simulink model "Ball_and_Plate_MicroLabBox_student"  (R2019b)
settings: Solver=ode1  StartTime=0.0  StopTime=Inf  FixedStep=0.001  RelTol=1e-3
PostLoadFcn:
  | , if any(exist('dsrtsu_mdlpostloadfcn', 'file') ~= 0), dsrtsu_mdlpostloadfcn('Execute', bdroot); end,
InitFcn:
  | , if any(exist('rtifpga_mdlclblib', 'file') ~= 0), rtifpga_mdlclblib('Init', bdroot); end,
values from neighbouring files (symbols this model uses):
  A_obs = A_fast - L*C_fast    [Init_workspace.m]
  B_obs = [B_fast, L]    [Init_workspace.m]
  C_obs = eye(4)    [Init_workspace.m]
  D_obs = zeros(4,4)    [Init_workspace.m]
  path = quintic(-0.0289,3,0,1/fs)    [Init_workspace.m]    (also in Quintic_Time.m = reference_end; Quintic_Velocity.m = reference_end)
  Ts_Outer = 0.1    [Init_workspace.m]
  uA = repmat(uA,[1,P])    [Init_workspace.m]
  uB = repmat(uB,[1,P])    [Init_workspace.m]
  uC = repmat(uC,[1,P])    [Init_workspace.m]
libraries: rtiemclib x6, rtiethernetlib x3, rti1202lib_dac_class1 x3, simulink x1
(part 3 of 3)

== matlab function Ball_and_Plate_MicroLabBox_student/Innerloop_Actuator/Motor_C/Init_motion/MATLAB Function1 ==
  data: reference_end input; path output; end_time input; Ts input; measured_position input
function path = Quintic_Polynomial_Trajectory_Time(reference_end, end_time, Ts, measured_position)
%% Quintic_Polynomial_Trajectory(reference_end, average_velocity)
% This function outputs a quintic polynomial trajectory over time in 
% Simulink given the end reference and average velocity. The starting 
% velocity and acceleration are set to zero.
%
% Input Arguments
% reference_end = desired end position of the trajectory
% end_time = end time of trajectory; for every new input 
% trajectory starts at time 0 and ends at end_time
% measured_position = current position of the robot arm
%
% Output Arguments
% path = path of the trajectory over time
%
% Quinten Swaan 17-08-2022
%
% Control Systems Technology group
% Departement of Mechanical Engineering
% Eindhoven University of Technology


persistent previous_value_reference_start previous_value_reference_end ...
    path_array index 

if isempty(previous_value_reference_start)
    previous_value_reference_start = 0;
end

if isempty(previous_value_reference_end)
    previous_value_reference_end = 0;
end

if isempty(path_array)
    path_array = zeros(1,1);
end

if isempty(index)
    index = 1;
end


% Obtain new trajectory if a new end reference is given
if previous_value_reference_end ~= reference_end
    t0 = 0;                                 %Starting time
    q0 = previous_value_reference_start;    %Starting position
    v0 = 0;                                 %Starting velocity
    ac0 = 0;                                %Starting acceleration
    tf = end_time;                          %End time
    qf = reference_end;                     %End position
    vf = 0;                                 %End velocity
    acf = 0;                                %End acceleration

    M = [1 t0 t0^2 t0^3 t0^4 t0^5;
    0 1 2*t0 3*t0^2 4*t0^3 5*t0^4;
    0 0 2 6*t0 12*t0^2 20*t0^3;
    1 tf tf^2 tf^3 tf^4 tf^5;
    0 1 2*tf 3*tf^2 4*tf^3 5*tf^4;
    0 0 2 6*tf 12*tf^2 20*tf^3];

    b = [q0; v0; ac0; qf; vf; acf];

    x = M \ b;

    t = t0:Ts:tf;

    path_array = x(1) + x(2).*t + x(3).*t.^2 + x(4).*t.^3 + +x(5).*t.^4 + x(6).*t.^5;

    index = 1;
    reference_current = path_array(index);

% Output the reference per timestep
else
    if index < length(path_array)
        index = index + 1;
    end
    reference_current = path_array(index);
end

previous_value_reference_end = reference_end;
previous_value_reference_start = measured_position;

path = reference_current;

== matlab function Ball_and_Plate_MicroLabBox_student/Innerloop_Actuator/Motor_C/Init_motion/MATLAB Function2 ==
  data: y input; path output; start input; init_value input; current_pos input
function path = init_motion(y, start, init_value, current_pos)

if start > 0.5
    path = init_value;
elseif start < 0.5
    path = y;
else 
    path = 0;
end

== matlab function Ball_and_Plate_MicroLabBox_student/Innerloop_Actuator/Motor_A/Init_motion/MATLAB Function ==
  data: enable input; u input; y output
function y = init_motion(enable, u)

persistent index previous_enable

% Initialize
if isempty(index)
    index = 1;
end

if isempty(previous_enable)
    previous_enable = 0;
end

N = length(u);

% Detect rising edge (re-enable)
if enable && ~previous_enable
    index = 1;
end

% Output logic
if enable

    % If still inside signal → output sample
    if index <= N
        y = u(index);
        index = index + 1;

    else
        % Signal finished → output zero
        y = 0;
    end

else
    % Disabled → output zero
    y = -0.0289;
end

previous_enable = enable;

== matlab function Ball_and_Plate_MicroLabBox_student/Innerloop_Actuator/Motor_B/Init_motion/MATLAB Function ==
  data: enable input; u input; y output
function y = init_motion(enable, u)

persistent index previous_enable

% Initialize
if isempty(index)
    index = 1;
end

if isempty(previous_enable)
    previous_enable = 0;
end

N = length(u);

% Detect rising edge (re-enable)
if enable && ~previous_enable
    index = 1;
end

% Output logic
if enable

    % If still inside signal → output sample
    if index <= N
        y = u(index);
        index = index + 1;

    else
        % Signal finished → output zero
        y = 0;
    end

else
    % Disabled → output zero
    y = -0.0289;
end

previous_enable = enable;

== matlab function Ball_and_Plate_MicroLabBox_student/Innerloop_Actuator/Motor_C/Init_motion/MATLAB Function ==
  data: enable input; u input; y output
function y = init_motion(enable, u)

persistent index previous_enable

% Initialize
if isempty(index)
    index = 1;
end

if isempty(previous_enable)
    previous_enable = 0;
end

N = length(u);

% Detect rising edge (re-enable)
if enable && ~previous_enable
    index = 1;
end

% Output logic
if enable

    % If still inside signal → output sample
    if index <= N
        y = u(index);
        index = index + 1;

    else
        % Signal finished → output zero
        y = 0;
    end

else
    % Disabled → output zero
    y = -0.0289;
end

previous_enable = enable;

== matlab function Ball_and_Plate_MicroLabBox_student/Innerloop_Actuator/AngleToPos  ==
  data: alpha input; pos1 output; beta input; psi input; pos2 output; pos3 output
function [pos1, pos2, pos3] = angleToPos(alpha, beta, psi)
    % Returns the actuator positions required to reach the desired angle
    % note: the position is absolute in the global frame

    % Physical Constants
    r = 0.17;           % Joint radius (m)
    T = [0; 0; 0.322];  % Resting height vector (m)
    
    % Joint positions on base and plate (equilateral triangle)
    % These match the definitions in your posToAngle function
    theta = [0, deg2rad(240), deg2rad(120)];
    B = [r*cos(theta); r*sin(theta); zeros(1,3)]; % Base joints (b_i)
    P = [r*cos(theta); r*sin(theta); zeros(1,3)]; % Plate joints (p_i)
    
    % Rotation Matrices (Yaw-Pitch-Roll order)
    Rz = [cos(psi) -sin(psi) 0; sin(psi) cos(psi) 0; 0 0 1];
    Ry = [cos(beta) 0 sin(beta); 0 1 0; -sin(beta) 0 cos(beta)];
    Rx = [1 0 0; 0 cos(alpha) -sin(alpha); 0 sin(alpha) cos(alpha)];
    R_BtoP = Rz * Ry * Rx; 
    
    % Compute absolute position for each motor
    % Motor 1
    l1_vec = T + (R_BtoP * P(:,1)) - B(:,1);
    pos1 = norm(l1_vec);
    
    % Motor 2
    l2_vec = T + (R_BtoP * P(:,2)) - B(:,2);
    pos2 = norm(l2_vec);
    
    % Motor 3
    l3_vec = T + (R_BtoP * P(:,3)) - B(:,3);
    pos3 = norm(l3_vec);
end

== matlab function Ball_and_Plate_MicroLabBox_student/Innerloop_Actuator/Motor_A/MATLAB Function1 ==
  data: reference_end input; path output; end_time input; Ts input; measured_position input
function path = Quintic_Time(reference_end, end_time, Ts, measured_position)
% QUINTIC_POLYNOMIAL_TRAJECTORY_TIME
% Calculated analytically per step to be compatible with dSPACE/Control Desk.

% Persistent variables to store coefficients and the "internal clock"
persistent coeffs t_elapsed prev_ref_end tf_internal
if isempty(coeffs)
    coeffs = zeros(6, 1); % a0, a1, a2, a3, a4, a5
end
if isempty(t_elapsed)
    t_elapsed = 0;
end
if isempty(prev_ref_end)
    prev_ref_end = reference_end;
end
if isempty(tf_internal)
    tf_internal = 0;
end

% Check if a new trajectory is requested
if reference_end ~= prev_ref_end
    % Reset timer
    t_elapsed = 0;
    tf_internal = end_time;
    
    % Boundary conditions
    q0 = prev_ref_end; 
    qf = reference_end;
    v0 = 0; vf = 0;
    ac0 = 0; acf = 0;
    
    % Solver for t0 = 0
    % We solve the system: M * coeffs = b
    % Using tf_internal instead of end_time to ensure consistency during the run
    T = tf_internal;
    M = [1, 0, 0,  0,    0,    0;
         0, 1, 0,  0,    0,    0;
         0, 0, 2,  0,    0,    0;
         1, T, T^2, T^3,  T^4,  T^5;
         0, 1, 2*T, 3*T^2, 4*T^3, 5*T^4;
         0, 0, 2,   6*T,   12*T^2, 20*T^3];
     
    b = [q0; v0; ac0; qf; vf; acf];
    
    % Calculate coefficients (Matrix is small 6x6, so this is fast)
    coeffs = M \ b;
end

% Calculate current reference based on elapsed time
t = t_elapsed;

if t <= tf_internal
    % Quintic Equation: path = a0 + a1*t + a2*t^2 + a3*t^3 + a4*t^4 + a5*t^5
    path = coeffs(1) + coeffs(2)*t + coeffs(3)*t^2 + coeffs(4)*t^3 + coeffs(5)*t^4 + coeffs(6)*t^5;
    
    % Increment time for the next step
    t_elapsed = t_elapsed + Ts;
else
    % Hold the final position once trajectory is finished
    path = reference_end;
end

% Update memory for next iteration
prev_ref_end = reference_end;

end

== matlab function Ball_and_Plate_MicroLabBox_student/Innerloop_Actuator/Motor_B/MATLAB Function2 ==
  data: reference_end input; path output; end_time input; Ts input; measured_position input
function path = Quintic_Time(reference_end, end_time, Ts, measured_position)
% QUINTIC_POLYNOMIAL_TRAJECTORY_TIME
% Calculated analytically per step to be compatible with dSPACE/Control Desk.

% Persistent variables to store coefficients and the "internal clock"
persistent coeffs t_elapsed prev_ref_end tf_internal
if isempty(coeffs)
    coeffs = zeros(6, 1); % a0, a1, a2, a3, a4, a5
end
if isempty(t_elapsed)
    t_elapsed = 0;
end
if isempty(prev_ref_end)
    prev_ref_end = reference_end;
end
if isempty(tf_internal)
    tf_internal = 0;
end

% Check if a new trajectory is requested
if reference_end ~= prev_ref_end
    % Reset timer
    t_elapsed = 0;
    tf_internal = end_time;
    
    % Boundary conditions
    q0 = prev_ref_end; 
    qf = reference_end;
    v0 = 0; vf = 0;
    ac0 = 0; acf = 0;
    
    % Solver for t0 = 0
    % We solve the system: M * coeffs = b
    % Using tf_internal instead of end_time to ensure consistency during the run
    T = tf_internal;
    M = [1, 0, 0,  0,    0,    0;
         0, 1, 0,  0,    0,    0;
         0, 0, 2,  0,    0,    0;
         1, T, T^2, T^3,  T^4,  T^5;
         0, 1, 2*T, 3*T^2, 4*T^3, 5*T^4;
         0, 0, 2,   6*T,   12*T^2, 20*T^3];
     
    b = [q0; v0; ac0; qf; vf; acf];
    
    % Calculate coefficients (Matrix is small 6x6, so this is fast)
    coeffs = M \ b;
end

% Calculate current reference based on elapsed time
t = t_elapsed;

if t <= tf_internal
    % Quintic Equation: path = a0 + a1*t + a2*t^2 + a3*t^3 + a4*t^4 + a5*t^5
    path = coeffs(1) + coeffs(2)*t + coeffs(3)*t^2 + coeffs(4)*t^3 + coeffs(5)*t^4 + coeffs(6)*t^5;
    
    % Increment time for the next step
    t_elapsed = t_elapsed + Ts;
else
    % Hold the final position once trajectory is finished
    path = reference_end;
end

% Update memory for next iteration
prev_ref_end = reference_end;

end

== matlab function Ball_and_Plate_MicroLabBox_student/Innerloop_Actuator/Motor_C/MATLAB Function1 ==
  data: reference_end input; path output; end_time input; Ts input; measured_position input
function path = Quintic_Time(reference_end, end_time, Ts, measured_position)
% QUINTIC_POLYNOMIAL_TRAJECTORY_TIME
% Calculated analytically per step to be compatible with dSPACE/Control Desk.

% Persistent variables to store coefficients and the "internal clock"
persistent coeffs t_elapsed prev_ref_end tf_internal
if isempty(coeffs)
    coeffs = zeros(6, 1); % a0, a1, a2, a3, a4, a5
end
if isempty(t_elapsed)
    t_elapsed = 0;
end
if isempty(prev_ref_end)
    prev_ref_end = reference_end;
end
if isempty(tf_internal)
    tf_internal = 0;
end

% Check if a new trajectory is requested
if reference_end ~= prev_ref_end
    % Reset timer
    t_elapsed = 0;
    tf_internal = end_time;
    
    % Boundary conditions
    q0 = prev_ref_end; 
    qf = reference_end;
    v0 = 0; vf = 0;
    ac0 = 0; acf = 0;
    
    % Solver for t0 = 0
    % We solve the system: M * coeffs = b
    % Using tf_internal instead of end_time to ensure consistency during the run
    T = tf_internal;
    M = [1, 0, 0,  0,    0,    0;
         0, 1, 0,  0,    0,    0;
         0, 0, 2,  0,    0,    0;
         1, T, T^2, T^3,  T^4,  T^5;
         0, 1, 2*T, 3*T^2, 4*T^3, 5*T^4;
         0, 0, 2,   6*T,   12*T^2, 20*T^3];
     
    b = [q0; v0; ac0; qf; vf; acf];
    
    % Calculate coefficients (Matrix is small 6x6, so this is fast)
    coeffs = M \ b;
end

% Calculate current reference based on elapsed time
t = t_elapsed;

if t <= tf_internal
    % Quintic Equation: path = a0 + a1*t + a2*t^2 + a3*t^3 + a4*t^4 + a5*t^5
    path = coeffs(1) + coeffs(2)*t + coeffs(3)*t^2 + coeffs(4)*t^3 + coeffs(5)*t^4 + coeffs(6)*t^5;
    
    % Increment time for the next step
    t_elapsed = t_elapsed + Ts;
else
    % Hold the final position once trajectory is finished
    path = reference_end;
end

% Update memory for next iteration
prev_ref_end = reference_end;

end

== matlab function Ball_and_Plate_MicroLabBox_student/Ethernet communication/MATLAB Function ==
  data: x output; u input; y output; z output
function [x,y,z] = fcn(u)
    x = double(u(9)) + 256*double(u(10));
    y = double(u(5)) + 256*double(u(6));
    z = double(u(1)) + 256*double(u(2));
    
    if x > 32767
        x = x-65536;
    end
    if y > 32767
        y = y-65536;
    end
    if z > 32767
        z = z-65536;
    end
%     if x_unsigned > 32767
%         x = double(x_unsigned) - 65536;
%     else
%         x = x_unsigned;
%     end
%     if y_unsigned > 32767
%         y = double(y_unsigned) - 65536;
%     else
%         y = y_unsigned;
%     end
%     if z_unsigned > 32767
%         z = double(z_unsigned) - 65536;
%     else
%         z = z_unsigned;
    end
